simulink model "Serial_Communication"  (R2020a)
settings: Solver=VariableStepAuto  StartTime=0.0  StopTime=inf  FixedStep=0.01  RelTol=1e-3
model workspace (MAT data in the model file):
  S = 1
undefined symbols (not defined in the file): serial
libraries: instrumentlib x3
settings Model: Creator=Vulca  LastModifiedBy=Vulca

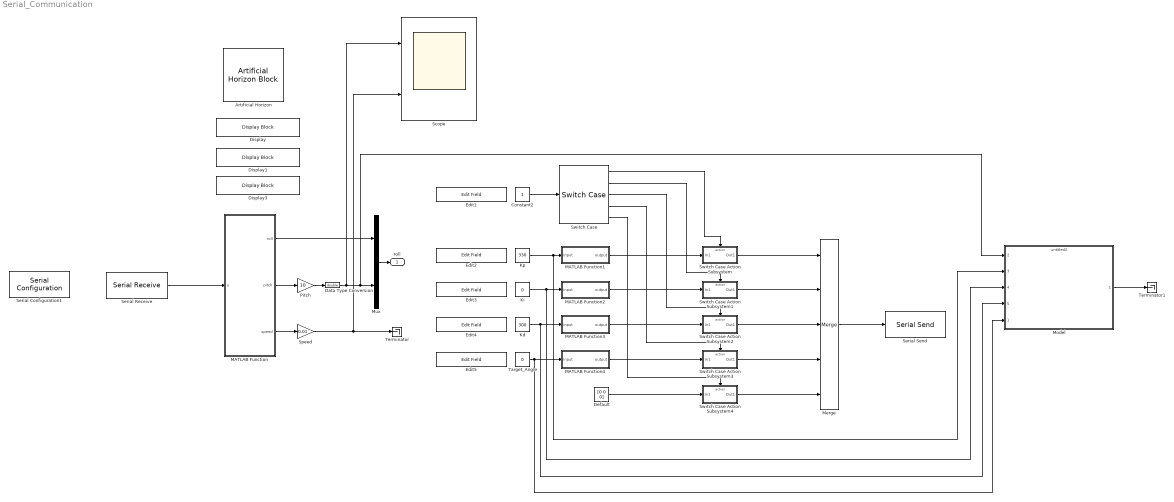
== system Serial_Communication ==
  Artificial Horizon : ArtificialHorizonBlock  LabelPosition=Bottom
  Constant2 : Constant
  Data Type Conversion : DataTypeConversion  OutDataTypeStr=double
  Default : Constant  Value=[0 0 0]  OutDataTypeStr=uint8  SampleTime=1
  Display : DisplayBlock  LabelPosition=Hide  Transparency=1
  Display1 : DisplayBlock  LabelPosition=Hide  Transparency=1
  Display3 : DisplayBlock  LabelPosition=Hide  Format=short  Transparency=1
  Edit{1..5} (5 alike) : EditField  LabelPosition=Hide  ShowInitialText=on  Alignment=Center
  Kd : Constant  Value=300  OutDataTypeStr=double  SampleTime=0.1
  Ki : Constant  Value=0  OutDataTypeStr=double  SampleTime=0.1
  Kp : Constant  Value=330  OutDataTypeStr=double  SampleTime=0.1
  MATLAB Function : MATLAB Function  TreatAsAtomicUnit=on
  MATLAB Function1 : MATLAB Function  TreatAsAtomicUnit=on
  MATLAB Function2 : MATLAB Function  TreatAsAtomicUnit=on
  MATLAB Function3 : MATLAB Function  TreatAsAtomicUnit=on
  MATLAB Function4 : MATLAB Function  TreatAsAtomicUnit=on
  Merge : Merge  Inputs=5  InitialOutput=[0 0 0]
  Model : ModelReference  ModelNameDialog=untitled2  SimulationMode=Normal  ModelReferenceVersion=1.37
      settings: PortSchema="{\"entries\":[{\"content\":{\"sides\":[{\"content\":{\"connectorIds\":[\"In2\",\"In3\",\"In4\",\"In5\",\"In1\"]},\"type\":\"ConnectorPlacement.EquallySpacedRectSide\",\"uuid\":\"b4f5d8f9-884c-41a8-9e96-95856cfa29c5\"},{\"content\":{\"connectorIds\":[\"Out1\"],\"side\":\"RIGHT\"},\"type\":\"ConnectorPlacement.EquallySpacedRectSide\",\"uuid\":\"52f3a4cf-e77c-4dc7-94d0-f162618e7e50\"},{\"content\":{\"connectorIds\":[],\"side\":\"TOP\"},\"type\":\"ConnectorPlacement.EquallySpacedRectSide\",\"uuid\":\"a60bd9fb-b553-4324-bdf5-90a3cfea07be\"}]},\"type\":\"ConnectorPlacement.EquallySpacedConnector\",\"uuid\":\"f4b9c641-306f-4d07-bcf8-3e214978a95c\"}],\"packageUris\":[\"http://schema.mathworks.com/mf0/Connector/19700101\"],\"version\":\"1.0\"}"
  Mux : Mux  Inputs=2
  Pitch : Gain  Gain=10
  Scope : Scope  NumInputPorts=2
  Serial Configuration1 : instrumentlib/Serial Configuration  Priority=-200000  ComPortMenu=<Please select a port...>  ComPort=COM12  ObjConstructor=serial('COM12');  BaudRate=115200  DataBits=8  Parity=none  StopBits=1  FlowControl=none  Timeout=10  ByteOrder=LittleEndian
  Serial Receive : instrumentlib/Serial Receive  ComPortMenu=<Please select a port...>  ComPort=COM12  ObjConstructor=serial('COM12');  Terminator=<none>  DataSize="[8  1]"  DataType=uint8  EnableBlockingMode=on  ActionDataUnavailable=Output last received value  CustomValue=0  SampleTime=0.01
  Serial Send : instrumentlib/Serial Send  ComPortMenu=<Please select a port...>  ComPort=COM12  ObjConstructor=serial('COM12');  Terminator=<none>  EnableBlockingMode=off
  Speed : Gain  Gain=0.01
  Switch Case : SwitchCase  CaseConditions={1,2,3,4}
  Switch Case Action Subsystem : Subsystem  TreatAsAtomicUnit=on
  Switch Case Action Subsystem1 : Subsystem  TreatAsAtomicUnit=on
  Switch Case Action Subsystem2 : Subsystem  TreatAsAtomicUnit=on
  Switch Case Action Subsystem3 : Subsystem  TreatAsAtomicUnit=on
  Switch Case Action Subsystem4 : Subsystem  TreatAsAtomicUnit=on
  Target_Angle : Constant  Value=0  OutDataTypeStr=double  SampleTime=0.1
  Terminator : Terminator
  Terminator1 : Terminator
  roll : Outport
  wires:
  Serial Receive/1 -> MATLAB Function/1(u)
  MATLAB Function/2(pitch) -> Pitch/1
  MATLAB Function/3(speed) -> Speed/1
  Speed/1 -> Terminator/1, Scope/2
  Mux/1 -> roll/1
  Data Type Conversion/1 -> Mux/2, Model/2, Scope/1
  MATLAB Function/1(roll) -> Mux/1
  Switch Case/1 -> Switch Case Action Subsystem/Action
  Switch Case/2 -> Switch Case Action Subsystem1/Action
  Switch Case/3 -> Switch Case Action Subsystem2/Action
  Switch Case/4 -> Switch Case Action Subsystem3/Action
  Switch Case/5 -> Switch Case Action Subsystem4/Action
  Constant2/1 -> Switch Case/1
  Switch Case Action Subsystem1/1(Out1) -> Merge/2
  Switch Case Action Subsystem2/1(Out1) -> Merge/3
  Switch Case Action Subsystem3/1(Out1) -> Merge/4
  Switch Case Action Subsystem4/1(Out1) -> Merge/5
  MATLAB Function1/1(output) -> Switch Case Action Subsystem/1(In1)
  Kp/1 -> Model/3, MATLAB Function1/1(input)
  Ki/1 -> MATLAB Function2/1(input), Model/4
  MATLAB Function2/1(output) -> Switch Case Action Subsystem1/1(In1)
  Kd/1 -> MATLAB Function3/1(input), Model/5
  MATLAB Function3/1(output) -> Switch Case Action Subsystem2/1(In1)
  Target_Angle/1 -> MATLAB Function4/1(input), Model/1
  MATLAB Function4/1(output) -> Switch Case Action Subsystem3/1(In1)
  Switch Case Action Subsystem/1(Out1) -> Merge/1
  Default/1 -> Switch Case Action Subsystem4/1(In1)
  Merge/1 -> Serial Send/1
  Model/1 -> Terminator1/1
  Pitch/1 -> Data Type Conversion/1

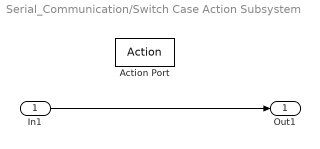
== system Serial_Communication/Switch Case Action Subsystem ==
  In1 : Inport
  Action Port : ActionPort  ActionPortLabel=case [ 1 ]:
  Out1 : Outport
  wires:
  In1/1 -> Out1/1

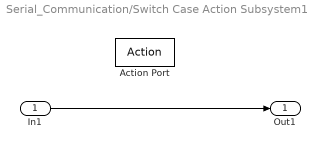
== system Serial_Communication/Switch Case Action Subsystem1 ==
  In1 : Inport
  Action Port : ActionPort  ActionPortLabel=case [ 2 ]:
  Out1 : Outport
  wires:
  In1/1 -> Out1/1

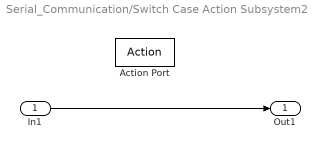
== system Serial_Communication/Switch Case Action Subsystem2 ==
  In1 : Inport
  Action Port : ActionPort  ActionPortLabel=case [ 3 ]:
  Out1 : Outport
  wires:
  In1/1 -> Out1/1

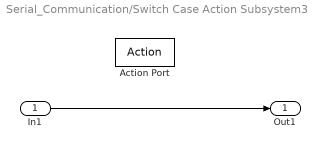
== system Serial_Communication/Switch Case Action Subsystem3 ==
  In1 : Inport
  Action Port : ActionPort  ActionPortLabel=case [ 4 ]:
  Out1 : Outport
  wires:
  In1/1 -> Out1/1

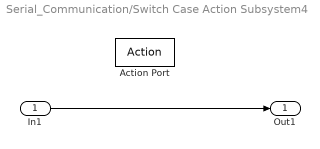
== system Serial_Communication/Switch Case Action Subsystem4 ==
  In1 : Inport
  Action Port : ActionPort  ActionPortLabel=default:
  Out1 : Outport
  wires:
  In1/1 -> Out1/1

== matlab function Serial_Communication/MATLAB Function1 ==
  data: output output; input input
function output= fcn(input)

int16 int16_input;
int16_input = input * 100;
int16_input = cast(int16_input,'int16');

int16 int16_input_H8;
int16 int16_input_L8;
int16_input_H8 = bitand(bitshift(int16_input,-8),cast(0xff,'int16'));
int16_input_L8 = bitand(int16_input,cast(0xff,'int16'));

output = zeros([1 3],'uint8');
output(1) =  0xA1;
output(2) =  int16_input_H8;
output(3) =  cast(int16_input_L8,'uint8');

== matlab function Serial_Communication/MATLAB Function ==
  data: roll output; u input; pitch output; speed output
function [roll,pitch,speed]= fcn(u)

int16 pitch;
pitchH = cast(u(2),'int16');
pitchL = cast(u(3),'int16');

int32 speed;
speedH24 = cast(u(4),'int32');
speedH16 = cast(u(5),'int32');
speedL8 = cast(u(6),'int32');
speedL = cast(u(7),'int32');

speedH16 =  bitor(bitshift(speedH24,8),speedH16);
speedL8 =  bitor(bitshift(speedH16,8),speedL8);

roll = 0;
pitch = bitor(bitshift(pitchH,8),pitchL);
speed = bitor(bitshift(speedL8,8),speedL);

== matlab function Serial_Communication/MATLAB Function2 ==
  data: output output; input input
function output= fcn(input)

int16 int16_input;
int16_input = input * 100;
int16_input = cast(int16_input,'int16');

int16 int16_input_H8;
int16 int16_input_L8;
int16_input_H8 = bitand(bitshift(int16_input,-8),cast(0xff,'int16'));
int16_input_L8 = bitand(int16_input,cast(0xff,'int16'));

output = zeros([1 3],'uint8');
output(1) =  0xA2;
output(2) =  int16_input_H8;
output(3) =  cast(int16_input_L8,'uint8');

== matlab function Serial_Communication/MATLAB Function3 ==
  data: output output; input input
function output= fcn(input)

int16 int16_input;
int16_input = input * 100;
int16_input = cast(int16_input,'int16');

int16 int16_input_H8;
int16 int16_input_L8;
int16_input_H8 = bitand(bitshift(int16_input,-8),cast(0xff,'int16'));
int16_input_L8 = bitand(int16_input,cast(0xff,'int16'));

output = zeros([1 3],'uint8');
output(1) =  0xA3;
output(2) =  int16_input_H8;
output(3) =  cast(int16_input_L8,'uint8');

== matlab function Serial_Communication/MATLAB Function4 ==
  data: output output; input input
function output= fcn(input)

int16 int16_input;
int16_input = input * 100;
int16_input = cast(int16_input,'int16');

int16 int16_input_H8;
int16 int16_input_L8;
int16_input_H8 = bitand(bitshift(int16_input,-8),cast(0xff,'int16'));
int16_input_L8 = bitand(int16_input,cast(0xff,'int16'));

output = zeros([1 3],'uint8');
output(1) =  0xA4;
output(2) =  int16_input_H8;
output(3) =  cast(int16_input_L8,'uint8');
